simulink subsystem "set_point"  (R2023b)
settings: Solver=VariableStepAuto  StartTime=0.0  StopTime=10.0  RelTol=1e-3
values from neighbouring files (symbols this model uses):
  r = 120    [constantes.m]
settings Model: Creator=Nahuel  LastModifiedBy=Nahuel

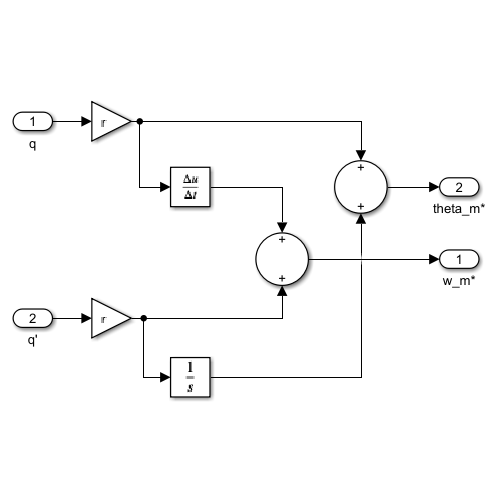
[thumbnail: Simulink's stored preview of the top-level diagram]
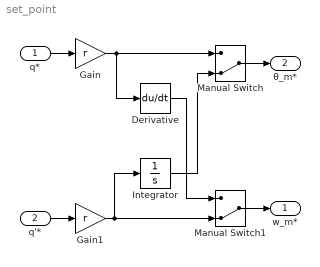
== system set_point ==
  q* : Inport
  q'* : Inport  Port=2
  Derivative : Derivative
  Gain : Gain  Gain=r
  Gain1 : Gain  Gain=r
  Integrator : Integrator
  Manual Switch : ManualSwitch  CurrentSetting=0
  Manual Switch1 : ManualSwitch  CurrentSetting=0
  w_m* : Outport
  θ_m* : Outport  Port=2
  wires:
  q*/1 -> Gain/1
  Gain/1 -> Manual Switch/1, Derivative/1
  q'*/1 -> Gain1/1
  Gain1/1 -> Manual Switch1/2, Integrator/1
  Integrator/1 -> Manual Switch/2
  Manual Switch/1 -> θ_m*/1
  Derivative/1 -> Manual Switch1/1
  Manual Switch1/1 -> w_m*/1
